simulink model "DAQ_PS"  (R2026a)
settings: Solver=FixedStepAuto  StopTime=inf  FixedStep=0.01  EnableMultiTasking=on
values from neighbouring files (symbols this model uses):
  Kg = 2.0    (= 2)    [MAAAAAAAAAAINNNNNN.m]
  Kt = 0.05667    [MAAAAAAAAAAINNNNNN.m]
  r = 0.006    [MAAAAAAAAAAINNNNNN.m]
  R_m = 3    [MAAAAAAAAAAINNNNNN.m]
  V_batt = 12    [MAAAAAAAAAAINNNNNN.m]
undefined symbols (not defined in the file or in its folder): K_rel
libraries: arduinolib x6, arduinosensorlib x1, slpidlib x1
settings Model: SimulationMode=external  SILPILModeSetting=veronly  ExtModeTrigDuration=2  Creator=Adham  LastModifiedBy=Adham
settings HardwareCC: ProdLargestAtomicInteger=Long  ProdLargestAtomicFloat=Double  ProdHWDeviceType=ARM Compatible->ARM Cortex  UseEmbeddedCoderFeatures=off
settings RTWCC: SystemTargetFile=ert.tlc  HardwareBoard=ESP32-WROOM (Arduino Compatible)  TLCOptions="-aInlineSetEventsForThisBaseRateFcn=TLC_FALSE -aSuppressMultiTaskScheduler=TLC_FALSE  -aRateBasedStepFcn=0"  Toolchain=ESP32  BuildConfiguration=Faster Runs  Description=Embedded Coder
settings RTWCC: CustomInclude=|
  | C:\ProgramData\MATLAB\SupportPackages\R2026a\aCLI\data\packages\esp32\hardware\esp32\2.0.17\libraries\Wire\src
  | D:\CoTune2026\Active_Suspension_resources\Parameter_Estimation_DAQ
  | D:\CoTune2026\Active_Suspension_resources\Parameter_Estimation_DAQ\core\inc
  | D:\CoTune2026\Active_Suspension_resources\Parameter_Estimation_DAQ\core\src
  | D:\CoTune2026\Active_Suspension_resources\Parameter_Estimation_DAQ\platform\inc
  | D:\CoTune2026\Active_Suspension_resources\Parameter_Estimation_DAQ\platform\src
settings RTWCC: CustomSource=|
  | C:\ProgramData\MATLAB\SupportPackages\R2026a\aCLI\data\packages\esp32\hardware\esp32\2.0.17\libraries\Wire\src\Wire.cpp
  | core\src\vl53l0x_api.cpp
  | core\src\vl53l0x_api_calibration.cpp
  | core\src\vl53l0x_api_core.cpp
  | core\src\vl53l0x_api_ranging.cpp
  | core\src\vl53l0x_api_strings.cpp
  | platform\src\vl53l0x_platform.cpp
  | Adafruit_VL53L0X.cpp
settings ERTTargetCC: ExtModeTransport=3.0  ExtModeAutomaticAllocSize=off  ExtModeStaticAllocSize=65536.0  SupportContinuousTime=on  SupportNonInlinedSFcns=on  SupportVariableSizeSignals=on

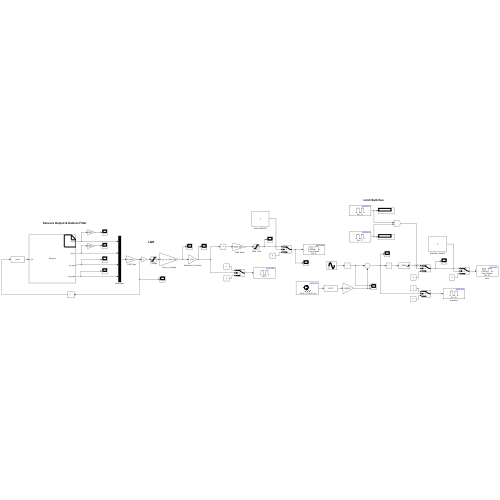
[thumbnail: Simulink's stored preview of the top-level diagram]
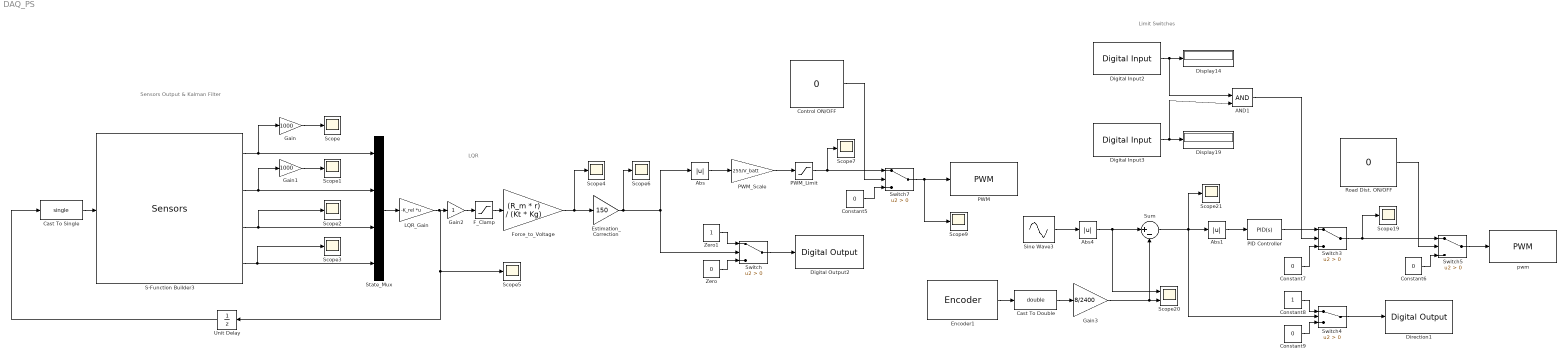
== system DAQ_PS ==
  note: Limit Switches
  note: Sensors Output & Kalman Filter
  note: LQR
  AND1 : Logic  IconShape=distinctive  AllPortsSameDT=off  OutDataTypeStr=boolean
  Abs : Abs  SaturateOnIntegerOverflow=off
  Abs1 : Abs  SaturateOnIntegerOverflow=off
  Abs4 : Abs  SaturateOnIntegerOverflow=off
  Cast To Double : DataTypeConversion  OutDataTypeStr=double  SaturateOnIntegerOverflow=off  RndMeth=Floor
  Cast To Single : DataTypeConversion  OutDataTypeStr=single  SaturateOnIntegerOverflow=off  RndMeth=Floor
  Constant{5..7,9} (4 alike) : Constant  Value=0
  Constant8 : Constant
  Control ON/OFF : Constant  Value=0
  Digital Input2 : arduinolib/Digital Input  pinNumber=16  mode=Input Pullup  Direction=input  SampleTime=0.1  blockPlatform=arduino
  Digital Input3 : arduinolib/Digital Input  pinNumber=17  mode=Input Pullup  Direction=input  SampleTime=0.1  blockPlatform=arduino
  Digital Output2 : arduinolib/Digital Output  pinNumber=4  Direction=output  blockPlatform=arduino
  Direction1 : arduinolib/Digital Output  pinNumber=18  Direction=output  blockPlatform=arduino
  Display14 : Display
  Display19 : Display
  Encoder1 : arduinosensorlib/Encoder  InputA=13  InputB=14  Mode=No reset  SampleTime=-1
  Estimation_Correction : Gain  Gain=150
  F_Clamp : Saturate  UpperLimit=10  LowerLimit=-10
  Force_to_Voltage : Gain  Gain=(R_m * r) / (Kt * Kg)
  Gain : Gain  Gain=1000
  Gain1 : Gain  Gain=1000
  Gain2 : Gain
  Gain3 : Gain  Gain=8/2400
  LQR_Gain : Gain  Gain=-K_rel  Multiplication=Matrix(K*u)
  PID Controller : slpidlib/PID Controller  Controller=PID  Form=Parallel  TimeDomain=Continuous-time  UseExternalTs=off  SampleTime=-1  IntegratorMethod=Forward Euler  FilterMethod=Forward Euler  ControllerParametersSource=internal  P=20  I=0  UseKiTs=off  D=0  UseExternalDerivativeSource=off  N=100  UseFilter=on  TunerSelectOption=Transfer Function Based (PID Tuner App)  InitialConditionSource=internal  InitialConditionForIntegrator=0  InitialConditionForFilter=0  DifferentiatorICPrevScaledInput=0  ExternalReset=none  TrackingMode=off  Kt=1  LimitOutput=on  SatLimitsSource=internal  UpperSaturationLimit=255  LowerSaturationLimit=-255  LinearizeAsGain=on  AntiWindupMode=none  Kb=1  LimitIntegrator=off  UpperIntegratorSaturationLimit=inf  LowerIntegratorSaturationLimit=-inf  POutMin=[]  POutMax=[]  IOutMin=[]  IOutMax=[]  DOutMin=[]  DOutMax=[]  NOutMin=[]  NOutMax=[]  SumOutMin=[]  SumOutMax=[]  SaturationOutMin=[]  SaturationOutMax=[]  PParamMin=[]  PParamMax=[]  IParamMin=[]  IParamMax=[]  DParamMin=[]  DParamMax=[]  NParamMin=[]  NParamMax=[]  KbParamMin=[]  KbParamMax=[]  KtParamMin=[]  KtParamMax=[]  KbOutMin=[]  KbOutMax=[]  KtOutMin=[]  KtOutMax=[]  IntegratorOutMin=[]  IntegratorOutMax=[]  FilterOutMin=[]  FilterOutMax=[]  SumI1OutMin=[]  SumI1OutMax=[]  SumI2OutMin=[]  SumI2OutMax=[]  SumI3OutMin=[]  SumI3OutMax=[]  SumI4OutMin=[]  SumI4OutMax=[]  SumDOutMin=[]  SumDOutMax=[]  DifferentiatorOutMin=[]  DifferentiatorOutMax=[]  FilterDiffOutCoefMin=[]  FilterDiffOutCoefMax=[]  ReciprocalOutMin=[]  ReciprocalOutMax=[]  SumDenOutMin=[]  SumDenOutMax=[]  SumNumOutMin=[]  SumNumOutMax=[]  DivideOutMin=[]  DivideOutMax=[]  UdiffTsProdOutMin=[]  UdiffTsProdOutMax=[]  NTsProdOutMin=[]  NTsProdOutMax=[]  UintegralTsProdOutMin=[]  UintegralTsProdOutMax=[]  UngainTsProdOutMin=[]  UngainTsProdOutMax=[]  ClampingZeroOutDataTypeStr=Inherit: Inherit via back propagation  ClampingZeroOutMin=[]  ClampingZeroOutMax=[]  FilterDenConstantOutDataTypeStr=Inherit: Inherit via back propagation  FilterDenConstantOutMin=[]  FilterDenConstantOutMax=[]  PCopyOutDataTypeStr=Inherit: Inherit via back propagation  PCopyOutMin=[]  PCopyOutMax=[]  NCopyOutDataTypeStr=Inherit: Inherit via back propagation  NCopyOutMin=[]  NCopyOutMax=[]  IntegratorContinuousStateAttributes=''  IntegratorStateMustResolveToSignalObject=off  IntegratorRTWStateStorageClass=Auto  FilterContinuousStateAttributes=''  FilterStateMustResolveToSignalObject=off  FilterRTWStateStorageClass=Auto  ParallelPVariant=InternalParameters  IdealPVariant=Disabled  IVariant=InternalParameters  DVariant=InternalParameters  IntegratorVariant=Continuous  SatVariant=Enabled  AWVariant=Passthrough  PCopyVariant=Disabled  TRVariant=Disabled  FdbkBlocksVariant=Forward  IdealPFdbkVariant=Disabled  SatFdbkVariant=Disabled  DerivativeFilterVariant=ContFilter  NVariant=InternalParameters  NCopyVariant=Disabled  FilterICVariant=InternalICsFilter  IntegratorICVariant=InternalICs  ExternalResetVariant=Disabled  TRSumVariant=Passthrough  SumFdbkVariant=Disabled  SumVariant=Sum_PID  TsampFilterVariant=InternalTs  TsampNgainVariant=Passthrough  TsampIntegralVariant=Disabled_SignalSpec  ExternalSaturationOutDataTypeStr=Inherit: Same as second input  DerivativeSourceVariant=ErrorSignal  PreIntVariant=InternalPreInt
  PWM : arduinolib/PWM  pinNumber=5  frequencyType=Default  desiredFrequency=490.2  achievableFrequency=490.2
  PWM_Limit : Saturate  UpperLimit=255  LowerLimit=0
  PWM_Scale : Gain  Gain=255/V_batt
  Road Dist. ON/OFF : Constant  Value=0
  S-Function Builder3 : S-Function  FunctionName=Sensors  SFunctionModules=Sensors_wrapper.cpp  SFunctionDeploymentMode=off  EnableBusSupport=off  mask(S-Function Builder){}
      mask help: Simulink:masks:SFunctionBuilder_MD
      mask init:
      | val = [[.9  0.75 0.75 1 1 .9 .9 1]',[1 1 0.75 0.75 .9 .9 1 .9]'];try , sys = get_param(gcb,'SfunBuilderFcnName');if isempty(sys), sys = get_param(gcb,'FunctionName'); end,catch, sys = get_param(gcb,'FunctionName'); end
      settings: CopyFcn=set_param(gcbh,'LinkStatus','none')  OpenFcn=sfunctionwizard(gcbh)
      mask Display:
      | plot(val(:,1),val(:,2))
      | disp(sys)
      | port_label('input',1,sprintf('%s', 'u\_N'),'interpreter','tex')
      | port_label('output',1,sprintf('%s', 'd1\_m'),'interpreter','tex')
      | port_label('output',2,sprintf('%s', 'd2\_m'),'interpreter','tex')
      | port_label('output',3,sprintf('%s', 'vs\_mps'),'interpreter','tex')
      | port_label('output',4,sprintf('%s', 'vus\_mps'),'interpreter','tex')
  Scope{,1..7,9,19,21} (11 alike) : Scope
      Scope settings: ActiveDisplayYMinimum=-6.3688507080078125  ActiveDisplayYMaximum=5.7446537017822266
      Scope1 settings: ActiveDisplayYMinimum=-10.222212970256805  ActiveDisplayYMaximum=15.830363929271698
      Scope19 settings: ActiveDisplayYMinimum=-19.129211768390523  ActiveDisplayYMaximum=172.16290591551473  DataLoggingVariableName=ScopeData21
      Scope2 settings: ActiveDisplayYMinimum=-0.27071841806173325  ActiveDisplayYMaximum=0.26262833923101425  DataLoggingVariableName=ScopeData2
      Scope21 settings: ActiveDisplayYMinimum=-49.886250000000004  ActiveDisplayYMaximum=49.54291666666667  DataLoggingVariableName=ScopeData23
      Scope3 settings: ActiveDisplayYMinimum=-0.35517418943345547  ActiveDisplayYMaximum=0.24406235478818417  DataLoggingVariableName=ScopeData3
      Scope4 settings: ActiveDisplayYMinimum=-1.9851773977279663  ActiveDisplayYMaximum=1.9851773977279663  DataLoggingVariableName=ScopeData4
      Scope5 settings: ActiveDisplayYMinimum=-0.20557155646383762  ActiveDisplayYMaximum=0.27836028672754765  DataLoggingVariableName=ScopeData5
      Scope6 settings: ActiveDisplayYMinimum=-0.030651113018393517  ActiveDisplayYMaximum=0.024268718436360359  DataLoggingVariableName=ScopeData6
      Scope7 settings: ActiveDisplayYMinimum=-18.64936136215692  ActiveDisplayYMaximum=167.87513655977091  DataLoggingVariableName=ScopeData7
      Scope9 settings: ActiveDisplayYMinimum=-14.369404100405514  ActiveDisplayYMaximum=129.33664663886884  DataLoggingVariableName=ScopeData9
  Scope20 : Scope  NumInputPorts=2
      settings: ActiveDisplayYMinimum=-7.4392770820519249  ActiveDisplayYMaximum=7.2142201736814382  DataLoggingVariableName=ScopeData22
  Sine Wave3 : Sin  Amplitude=25  Frequency=15  SampleTime=0
  State_Mux : Mux
  Sum : Sum  Inputs=|+-
  Switch{,3..5,7} (5 alike) : Switch  Criteria=u2 > Threshold  SaturateOnIntegerOverflow=off  InputSameDT=off
  Unit Delay : UnitDelay  SampleTime=-1
  Zero : Constant  Value=0
  Zero1 : Constant
  pwm : arduinolib/PWM  pinNumber=19  frequencyType=Default  desiredFrequency=490.2  achievableFrequency=490.2
  wires:
  Digital Input3/1 -> AND1/2, Display19/1
  Sum/1 -> Scope21/1, Switch4/2, Abs1/1
  AND1/1 -> Switch3/2
  Constant7/1 -> Switch3/3
  Switch3/1 -> Scope19/1, Switch5/1
  Switch4/1 -> Direction1/1
  Constant9/1 -> Switch4/3
  Constant8/1 -> Switch4/1
  Abs1/1 -> PID Controller/1
  Digital Input2/1 -> AND1/1, Display14/1
  Sine Wave3/1 -> Abs4/1
  Gain3/1 -> Sum/2, Scope20/2
  PID Controller/1 -> Switch3/1
  Road Dist. ON/OFF/1 -> Switch5/2
  Constant6/1 -> Switch5/3
  Switch5/1 -> pwm/1
  Encoder1/1 -> Cast To Double/1
  Cast To Double/1 -> Gain3/1
  Zero1/1 -> Switch/1
  Switch/1 -> Digital Output2/1
  PWM_Scale/1 -> PWM_Limit/1
  Abs/1 -> PWM_Scale/1
  Force_to_Voltage/1 -> Scope4/1, Estimation_Correction/1
  PWM_Limit/1 -> Scope7/1, Switch7/1
  State_Mux/1 -> LQR_Gain/1
  Zero/1 -> Switch/3
  Switch7/1 -> PWM/1, Scope9/1
  Control ON/OFF/1 -> Switch7/2
  Constant5/1 -> Switch7/3
  Abs4/1 -> Sum/1, Scope20/1
  LQR_Gain/1 -> Scope5/1, Unit Delay/1, Gain2/1
  Cast To Single/1 -> S-Function Builder3/1
  Gain/1 -> Scope/1
  Gain1/1 -> Scope1/1
  S-Function Builder3/3 -> State_Mux/3, Scope2/1
  S-Function Builder3/4 -> State_Mux/4, Scope3/1
  S-Function Builder3/1 -> State_Mux/1, Gain/1
  S-Function Builder3/2 -> State_Mux/2, Gain1/1
  F_Clamp/1 -> Force_to_Voltage/1
  Unit Delay/1 -> Cast To Single/1
  Estimation_Correction/1 -> Abs/1, Switch/2, Scope6/1
  Gain2/1 -> F_Clamp/1
